simulink model "multibody_model"  (R2026a)
settings: Solver=ode14x  StopTime=10  FixedStep=0.0001
PreLoadFcn:
  | Dpx = Simulink.Parameter; Dpx.Value = 1E-6; Dpx.CoderInfo.StorageClass = 'ExportedGlobal';
  | Ipx = Simulink.Parameter; Ipx.Value = 1E-6; Ipx.CoderInfo.StorageClass = 'ExportedGlobal';
  | Npx = Simulink.Parameter; Npx.Value = 65;   Npx.CoderInfo.StorageClass = 'ExportedGlobal';
  | Ppx = Simulink.Parameter; Ppx.Value = 300;  Ppx.CoderInfo.StorageClass = 'ExportedGlobal';
  | Dvx = Simulink.Parameter; Dvx.Value = 1E-6; Dpx.CoderInfo.StorageClass = 'ExportedGlobal';
  | Ivx = Simulink.Parameter; Ivx.Value = 1E-6; Ipx.CoderInfo.StorageClass = 'ExportedGlobal';
  | Nvx = Simulink.Parameter; Nvx.Value = 65;   Npx.CoderInfo.StorageClass = 'ExportedGlobal';
  | Pvx = Simulink.Parameter; Pvx.Value = 300;  Ppx.CoderInfo.StorageClass = 'ExportedGlobal';
  | 
  | Dpy = Simulink.Parameter; Dpy.Value = 1E-6; Dpx.CoderInfo.StorageClass = 'ExportedGlobal';
  | Ipy = Simulink.Parameter; Ipy.Value = 1E-6; Ipx.CoderInfo.StorageClass = 'ExportedGlobal';
  | Npy = Simulink.Parameter; Npy.Value = 65;   Npx.CoderInfo.StorageClass = 'ExportedGlobal';
  | Ppy = Simulink.Parameter; Ppy.Value = 300;  Ppx.CoderInfo.StorageClass = 'ExportedGlobal';
  | Dvy = Simulink.Parameter; Dvy.Value = 1E-6; Dpx.CoderInfo.StorageClass = 'ExportedGlobal';
  | Ivy = Simulink.Parameter; Ivy.Value = 1E-6; Ipx.CoderInfo.StorageClass = 'ExportedGlobal';
  | Nvy = Simulink.Parameter; Nvy.Value = 65;   Npx.CoderInfo.StorageClass = 'ExportedGlobal';
  | Pvy = Simulink.Parameter; Pvy.Value = 300;  Ppx.CoderInfo.StorageClass = 'ExportedGlobal';
  | 
  | Dz = Simulink.Parameter; Dz.Value = 1E-6; Dpx.CoderInfo.StorageClass = 'ExportedGlobal';
  | Iz = Simulink.Parameter; Iz.Value = 1E-6; Ipx.CoderInfo.StorageClass = 'ExportedGlobal';
  | Nz = Simulink.Parameter; Nz.Value = 65;   Npx.CoderInfo.StorageClass = 'ExportedGlobal';
  | Pz = Simulink.Parameter; Pz.Value = 300;  Ppx.CoderInfo.StorageClass = 'ExportedGlobal';
  | 
  | Da = Simulink.Parameter; Da.Value = 1E-6; Dpx.CoderInfo.StorageClass = 'ExportedGlobal';
  | Ia = Simulink.Parameter; Ia.Value = 1E-6; Ipx.CoderInfo.StorageClass = 'ExportedGlobal';
  | Na = Simulink.Parameter; Na.Value = 65;   Npx.CoderInfo.StorageClass = 'ExportedGlobal';
  | Pa = Simulink.Parameter; Pa.Value = 300;  Ppx.CoderInfo.StorageClass = 'ExportedGlobal';
  | 
  | Dc = Simulink.Parameter; Dc.Value = 1E-6; Dpx.CoderInfo.StorageClass = 'ExportedGlobal';
  | Ic = Simulink.Parameter; Ic.Value = 1E-6; Ipx.CoderInfo.StorageClass = 'ExportedGlobal';
  | Nc = Simulink.Parameter; Nc.Value = 65;   Npx.CoderInfo.StorageClass = 'ExportedGlobal';
  | Pc = Simulink.Parameter; PcValue = 300;  Ppx.CoderInfo.StorageClass = 'ExportedGlobal';
settings Model: Creator=leo  LastModifiedBy=leo
settings SimscapeCC: SimscapeNominalValues="[{\"value\":\"1\",\"unit\":\"A\"},{\"value\":\"1\",\"unit\":\"bar\"},{\"value\":\"1\",\"unit\":\"cm^2\"},{\"value\":\"1\",\"unit\":\"cm^3/s\"},{\"value\":\"1\",\"unit\":\"kJ/kg\"},{\"value\":\"1\",\"unit\":\"kW\"},{\"value\":\"1\",\"unit\":\"l\"},{\"value\":\"1\",\"unit\":\"N\"},{\"value\":\"1\",\"unit\":\"N*m\"},{\"value\":\"1\",\"unit\":\"V\"}]"  SimscapeLogType=none  SimscapeLogDataHistory=5000.0

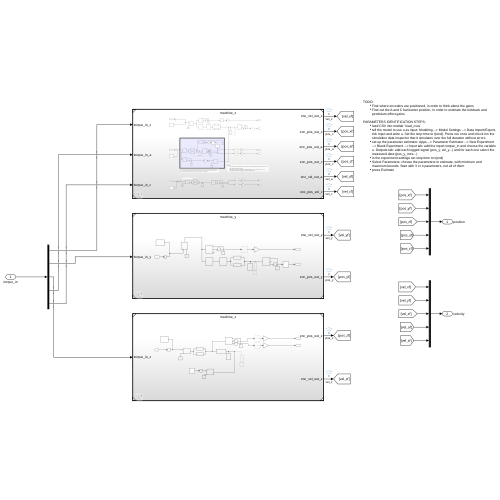
[thumbnail: Simulink's stored preview of the top-level diagram]
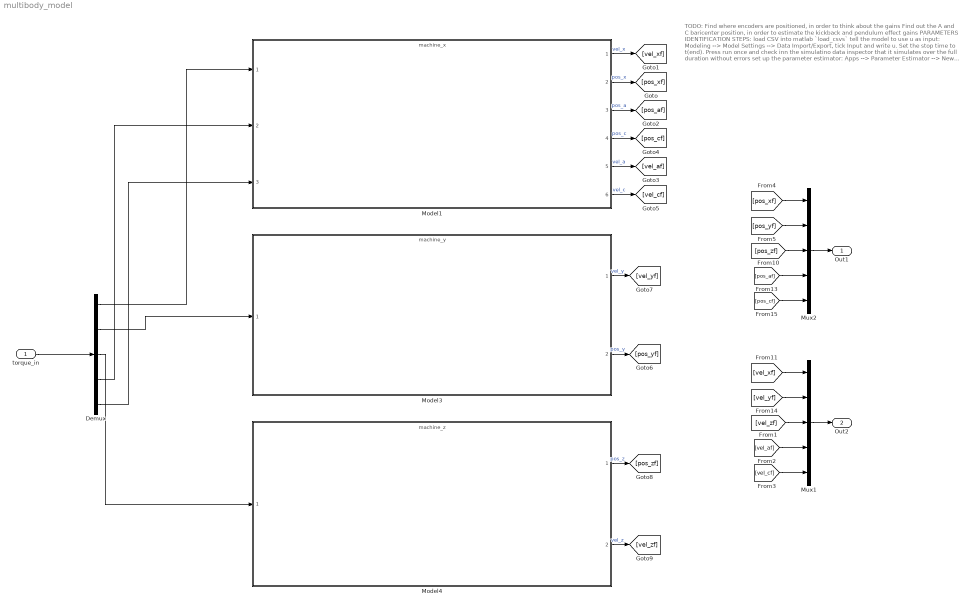
== system multibody_model ==
  note: TODO:
      | Find where encoders are positioned, in order to think about the gains
      | Find out the A and C baricenter position, in order to estimate the kickback and pendulum effect gains
      |
      | PARAMETERS IDENTIFICATION STEPS:
      | load CSV into matlab `load_csvs`
      | tell the model to use u as input: Modeling --> Model Settings --> Data Import/Export, tick Input and write u. Set the stop time to t(end). Press run once and check inn the simulatino data inspector that it simulates over the full duration without errors
      | set up the parameter estimator: Apps --> Parameter Estimator --> New Experiment --> Blank Experiment --> Input tab: add the inport torque_in and choose the variable u. Outputs tab: add each logged signal (pos_y, vel_y...) and for each one select the measured data (pos_y_mes...)
      | in the experiment settings set stop time to t(end)
      | Select Parameters: choose the parameters to estimate, with minimum and maximum bounds. Start with 3 or 4 parameters, not all of them
      | press Estimate
  torque_in : Inport
  Demux : Demux  Outputs=5
  Model1 : ModelReference  ModelNameDialog=machine_x.slx  SimulationMode=Normal  ModelReferenceVersion=2.10
  Model3 : ModelReference  ModelNameDialog=machine_y.slx  SimulationMode=Normal  ModelReferenceVersion=2.5
  Model4 : ModelReference  ModelNameDialog=machine_z.slx  SimulationMode=Normal  ModelReferenceVersion=2.5
  Mux1 : Mux  Inputs=5
  Mux2 : Mux  Inputs=5
  Out1 : Outport  SignalName=position
  Out2 : Outport  Port=2  SignalName=velocity
  wires:
  [pos_xf] -> Mux2/1
  [pos_yf] -> Mux2/2
  [pos_zf] -> Mux2/3
  [pos_af] -> Mux2/4
  [pos_cf] -> Mux2/5
  Mux2/1 -> Out1/1
  torque_in/1 -> Demux/1
  Demux/1 -> Model1/1
  Demux/2 -> Model3/1
  Demux/3 -> Model4/1
  Demux/4 -> Model1/2
  Demux/5 -> Model1/3
  [vel_af] -> Mux1/4
  Mux1/1 -> Out2/1
  [vel_yf] -> Mux1/2
  [vel_zf] -> Mux1/3
  [vel_xf] -> Mux1/1
  [vel_cf] -> Mux1/5
  Model1/2 -> [pos_xf]  "pos_x"
  Model1/1 -> [vel_xf]  "vel_x"
  Model1/3 -> [pos_af]  "pos_a"
  Model1/4 -> [pos_cf]  "pos_c"
  Model1/5 -> [vel_af]  "vel_a"
  Model1/6 -> [vel_cf]  "vel_c"
  Model3/1 -> [vel_yf]  "vel_y"
  Model3/2 -> [pos_yf]  "pos_y"
  Model4/1 -> [pos_zf]  "pos_z"
  Model4/2 -> [vel_zf]  "vel_z"
